simulink model "sldrt"  (R2018b)
settings: Solver=FixedStepAuto  StartTime=0.0  StopTime=Inf  FixedStep=1  RelTol=1e-3  EnableMultiTasking=on
values from neighbouring files (symbols this model uses):
  cpw = 4175    [symulacja.m]
  Cv01 = cpw*row*Vv    (= 801600)    [symulacja.m]
  Cv02 = cpw*row*Vv    (= 801600)    [symulacja.m]
  Cvg1 = cpw*row*Vg1    (= 400800)    [symulacja.m]
  Cvg2 = cpw*row*Vg2    (= 400800)    [symulacja.m]
  Cvs1 = cps*ros*Vs1    (= 38412000)    [symulacja.m]
  Cvs2 = cps*ros*Vs2    (= 38412000)    [symulacja.m]
  Cvw1 = cpp*rop*Vw1    (= 60000)    [symulacja.m]
  Cvw2 = cpp*rop*Vw2    (= 60000)    [symulacja.m]
  dfmw = 0    [symulacja.m]
  dTwz = 0    [symulacja.m]
  dTzew = 0    [symulacja.m]
  fmg1_0 = fmg1_N    (= 0.0239520958084)    [symulacja.m]
  fmg2_0 = fmg2_N    (= 0.0239520958084)    [symulacja.m]
  fmw0 = fmwN    (= 0.0479041916168)    [symulacja.m]
  Kcg1 = qg1_N/(Tgp1_N-Twew1_N)    (= 40)    [symulacja.m]
  Kcg2 = qg2_N/(Tgp2_N-Twew2_N)    (= 38.4615384615)    [symulacja.m]
  Kco = qwN/(TwpN-TozN)    (= 200)    [symulacja.m]
  Kcs1 = qg1_N/(Ts1_N-TzewN)    (= 80)    [symulacja.m]
  Kcs2 = qg2_N/(Ts2_N-TzewN)    (= 83.3333333333)    [symulacja.m]
  Kcw1 = qg1_N/(Twew1_N-Ts1_N)    (= 133.333333333)    [symulacja.m]
  Kcw2 = qg2_N/(Twew2_N-Ts2_N)    (= 142.857142857)    [symulacja.m]
  steptime = 1*czas/10^2    (= 30000)    [symulacja.m]
  Tdelay1 = 16000    [symulacja.m]
  Tdelay2 = Tdelay1    (= 16000)    [symulacja.m]
  Tgp1_0 = (C_1*Tgz1_0+Kcg1*Twew1_0)/(Kcg1+C_1)    (= 70)    [symulacja.m]
  Tgp2_0 = (C_2*Tgz2_0+Kcg2*Twew2_0)/(Kcg2+C_2)    (= 70)    [symulacja.m]
  Toz0 = (Kco*C1*Twz0+C2*(C1+Kco)*Top0)/M_1    (= 90)    [symulacja.m]
  Ts1_0 = (Kcw1*Twew1_0+Kcs1*Tzew0)/(Kcw1+Kcs1)    (= 5)    [symulacja.m]
  Ts2_0 = (Kcw2*Twew2_0+Kcs2*Tzew0)/(Kcw2+Kcs2)    (= 4)    [symulacja.m]
  Twew1_0 = (Kcg1*C_1*(Kcw1+Kcs1)*Tgz1_0+Kcw1*Kcs1*(Kcg1+C_1)*Tzew0)/M_1    (= 20)    [symulacja.m]
  Twew2_0 = (Kcg2*C_2*(Kcw2+Kcs2)*Tgz2_0+Kcw2*Kcs2*(Kcg2+C_2)*Tzew0)/M_2    (= 18)    [symulacja.m]
  Twp0 = (C1*Twz0+Kco*Toz0)/(C1+Kco)    (= 110)    [symulacja.m]
  Twz0 = TwzN    (= 130)    [symulacja.m]
  Tzew0 = TzewN    (= -20)    [symulacja.m]
libraries: sldrtlib x1
Description:
  | Water Tank Model with Dashboard
  | 
  | The example model "sldrtex_dashboard" shows a real-time model of a water tank
  | controlled by dashboard controls.  You can change the inputs to the plant using
  | the knobs and observe the response on the gauges.
  | 
  | How to run this model in Normal Mode:
  | 
  | 1) Double-click the orange button to switch to Normal Mode if needed.
  | 2) Start the real-time execution using Simulation->Run.
  | 3) Change the input flow and output valve values by the dashboard controls and observe
  |    the results on the dashboard gauges.
  | 
  | How to run this model in External Mode:
  | 
  | 1) Double-click the orange button to switch to External Mode if needed.
  | 2) Start the real-time execution using Simulation->Run. The model will automatically
  |    build, connect to Simulink in External Mode and start.
  | 3) Change the input flow and output valve values by the dashboard controls and observe
  |    the results on the dashboard gauges.
settings Model: EnablePacing=on  PacingRate=8000  ExtModeTrigDuration=101  Creator=The MathWorks, Inc.  LastModifiedBy=r3vus
settings DataIOCC: LimitDataPoints=on  SaveFormat=Array  SignalLoggingName=logsOut
settings OptimizationCC: ExpressionDepthLimit=2147483647  InitFltsAndDblsToZero=on  EfficientMapNaN2IntZero=off  LifeSpan=inf
settings DebuggingCC: UnderspecifiedInitializationDetection=Classic  MergeDetectMultiDrivingBlocksExec=none  SignalResolutionControl=TryResolveAllWithWarning  FcnCallInpInsideContextMsg=warning  AllowSymbolicDim=off  StateNameClashWarn=warning  SFUnexpectedBacktrackingDiag=warning  SFNoUnconditionalDefaultTransitionDiag=warning  SFExecutionAtInitializationDiag=none
settings HardwareCC: TargetBitPerLong=64  TargetBitPerPointer=64  TargetBitPerSizeT=64  TargetBitPerPtrDiffT=64  TargetIntDivRoundTo=Zero  TargetEndianess=LittleEndian  TargetWordSize=64  TargetHWDeviceType=Intel->x86-64
settings ModelReferenceCC: PropagateSignalLabelsOutOfModel=off
settings SFSimCC: SimUseLocalCustomCode=off
settings RTWCC: SystemTargetFile=sldrt.tlc  TemplateMakefile=sldrt.tmf  Description=Simulink Desktop Real-Time  RTWUseLocalCustomCode=off  RTWCompilerOptimization=on
settings CodeAppCC: MaxIdLength=95  StateflowObjectComments=on
settings SimulinkDesktopRealTimeCC: TargetPreCompLibLocation=D:\Program Files\MATLAB\R2018b\toolbox\sldrt\lib\win64  TargetLangStandard=C89/C90 (ANSI)  GeneratePreprocessorConditionals=Disable all  SupportVariableSizeSignals=off  PreserveStateflowLocalDataDimensions=off
settings ConfigComp: CovMetricSettings=dw  CovHtmlReporting=on  CovSaveCumulativeToWorkspaceVar=on  CovSaveSingleToWorkspaceVar=on  CovShowResultsExplorer=off  CovExternalEMLEnable=off  CovSFcnEnable=off

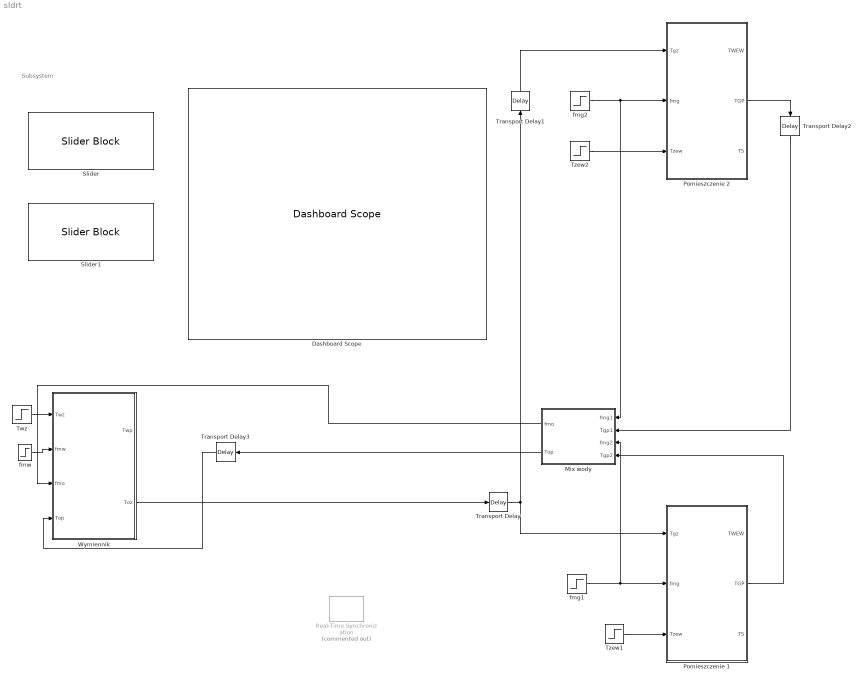
== system sldrt ==
  note: Subsystem
  Dashboard Scope : DashboardScope  WebBlockId=55  Ymin=10  Ymax=50
  Mix wody : Subsystem
  Pomieszczenie 1 : Subsystem  mask{Cvg=Cvg1, Cvs=Cvs1, Kcg=Kcg1, Kcw=Kcw1, cpw=cpw, Kcs=Kcs1, Cvw=Cvw1, Twew0=Twew1_0, Ts0=Ts1_0, Tgp0=Tgp1_0}
  Pomieszczenie 2 : Subsystem  mask{Cvg=Cvg2, Cvs=Cvs2, Kcg=Kcg2, Kcw=Kcw2, cpw=cpw, Kcs=Kcs2, Cvw=Cvw2, Twew0=Twew2_0, Ts0=Ts2_0, Tgp0=Tgp2_0}
  Real-Time Synchronization : sldrtlib/Real-Time Synchronization  Commented=on  SampleTime=1  MaxMissedTicks=10  ShowMissedTicks=off  YieldWhenWaiting=off
  Slider : SliderBlock  WebBlockId=118  ScaleMin=-20  ScaleMax=30
  Slider1 : SliderBlock  WebBlockId=119  ScaleMin=100  ScaleMax=130
  Transport Delay : TransportDelay  DelayTime=Tdelay1  InitialOutput=Toz0
  Transport Delay1 : TransportDelay  DelayTime=Tdelay2  InitialOutput=Toz0
  Transport Delay2 : TransportDelay  DelayTime=Tdelay2  InitialOutput=Tgp2_0
  Transport Delay3 : TransportDelay  DelayTime=Tdelay1  InitialOutput=(Tgp1_0*fmg1_0+Tgp2_0*fmg2_0)/(fmg1_0+fmg2_0)
  Twz : Step  Time=steptime  Before=Twz0  After=Twz0+dTwz  SampleTime=0
  Tzew1 : Step  Time=steptime  Before=Tzew0  After=Tzew0+dTzew  SampleTime=0
  Tzew2 : Step  Time=steptime  Before=Tzew0  After=Tzew0+dTzew  SampleTime=0
  Wymiennik : Subsystem
  fmg1 : Step  Time=steptime  Before=fmg1_0  After=fmg1_0  SampleTime=0
  fmg2 : Step  Time=steptime  Before=fmg2_0  After=fmg2_0  SampleTime=0
  fmw : Step  Time=steptime  Before=fmw0  After=fmw0+dfmw  SampleTime=0
  wires:
  Transport Delay1/1 -> Pomieszczenie 2/1(Tgz)
  Transport Delay3/1 -> Wymiennik/4(Top)
  Pomieszczenie 2/2(TGP) -> Transport Delay2/1
  Mix wody/1(fmo) -> Wymiennik/3(fmo)
  Transport Delay/1 -> Pomieszczenie 1/1(Tgz), Transport Delay1/1
  Mix wody/2(Top) -> Transport Delay3/1
  Wymiennik/2(Toz) -> Transport Delay/1
  fmg2/1 -> Mix wody/1(fmg1), Pomieszczenie 2/2(fmg)
  Twz/1 -> Wymiennik/1(Twz)
  Tzew1/1 -> Pomieszczenie 1/3(Tzew)
  Pomieszczenie 1/2(TGP) -> Mix wody/4(Tgp2)
  fmg1/1 -> Mix wody/3(fmg2), Pomieszczenie 1/2(fmg)
  Tzew2/1 -> Pomieszczenie 2/3(Tzew)
  fmw/1 -> Wymiennik/2(fmw)
  Transport Delay2/1 -> Mix wody/2(Tgp1)

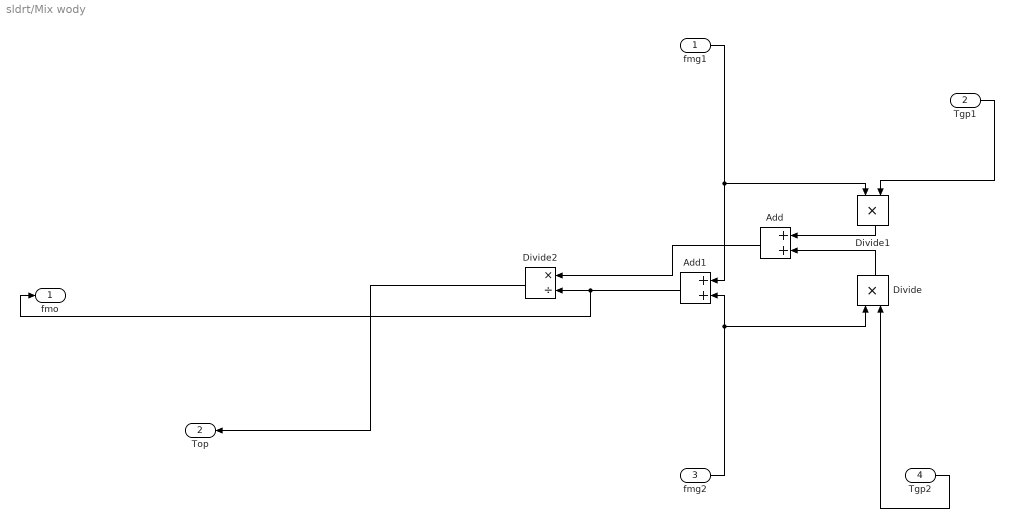
== system sldrt/Mix wody ==
  fmg1 : Inport
  Tgp1 : Inport  Port=2
  fmg2 : Inport  Port=3
  Tgp2 : Inport  Port=4
  Add : Sum
  Add1 : Sum
  Divide : Product  Inputs=**
  Divide1 : Product  Inputs=**
  Divide2 : Product  Inputs=*/
  fmo : Outport
  Top : Outport  Port=2
  wires:
  Tgp1/1 -> Divide1/2
  fmg2/1 -> Add1/2, Divide/1
  Divide/1 -> Add/2
  Add1/1 -> fmo/1, Divide2/2
  Tgp2/1 -> Divide/2
  fmg1/1 -> Add1/1, Divide1/1
  Divide1/1 -> Add/1
  Add/1 -> Divide2/1
  Divide2/1 -> Top/1

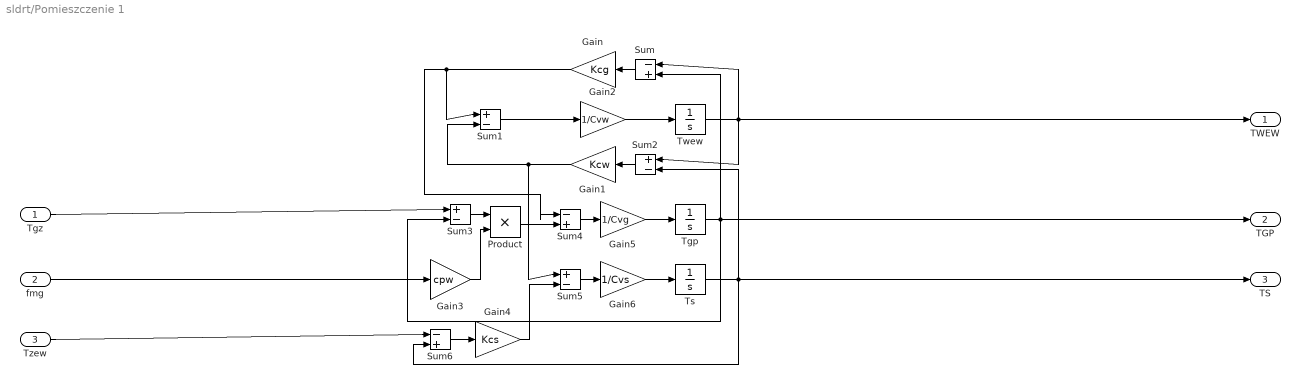
== system sldrt/Pomieszczenie 1 ==
  Tgz : Inport
  fmg : Inport  Port=2
  Tzew : Inport  Port=3
  Gain : Gain  Gain=Kcg
  Gain1 : Gain  Gain=Kcw
  Gain2 : Gain  Gain=1/Cvw
  Gain3 : Gain  Gain=cpw
  Gain4 : Gain  Gain=Kcs
  Gain5 : Gain  Gain=1/Cvg
  Gain6 : Gain  Gain=1/Cvs
  Product : Product
  Sum : Sum  Inputs=|-+
  Sum{1..3,5} (4 alike) : Sum  Inputs=|+-
  Sum4 : Sum  Inputs=|-+
  Sum6 : Sum  Inputs=|-+
  Tgp : Integrator  InitialCondition=Tgp0
  Ts : Integrator  InitialCondition=Ts0
  Twew : Integrator  InitialCondition=Twew0
  TWEW : Outport
  TGP : Outport  Port=2
  TS : Outport  Port=3
  wires:
  Twew/1 -> TWEW/1, Sum2/1, Sum/1
  Tgp/1 -> TGP/1, Sum3/2, Sum/2
  Sum/1 -> Gain/1
  Ts/1 -> TS/1, Sum6/2, Sum2/2
  Sum2/1 -> Gain1/1
  Gain1/1 -> Sum5/1, Sum1/2
  Sum1/1 -> Gain2/1
  Tgz/1 -> Sum3/1
  fmg/1 -> Gain3/1
  Gain3/1 -> Product/2
  Sum3/1 -> Product/1
  Gain/1 -> Sum1/1, Sum4/1
  Product/1 -> Sum4/2
  Sum4/1 -> Gain5/1
  Tzew/1 -> Sum6/1
  Sum6/1 -> Gain4/1
  Gain4/1 -> Sum5/2
  Sum5/1 -> Gain6/1
  Gain2/1 -> Twew/1
  Gain5/1 -> Tgp/1
  Gain6/1 -> Ts/1

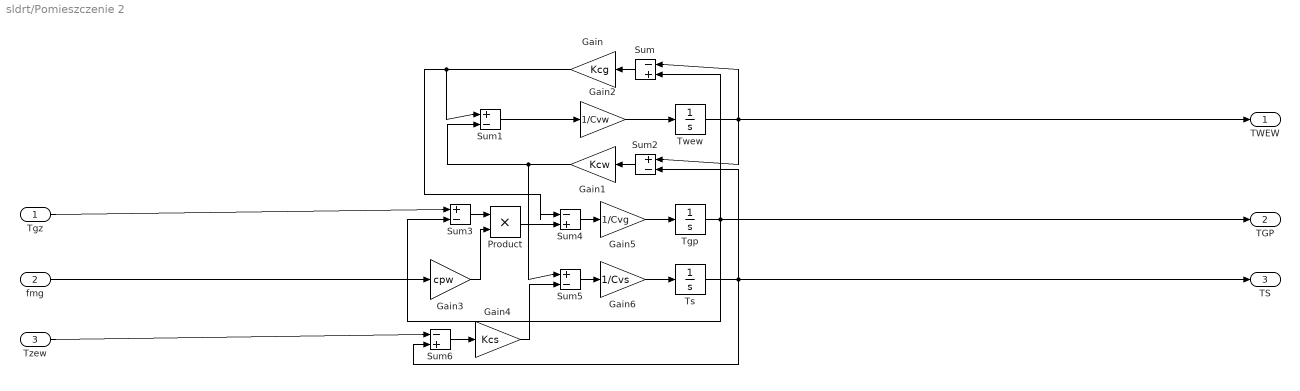
== system sldrt/Pomieszczenie 2 ==
  Tgz : Inport
  fmg : Inport  Port=2
  Tzew : Inport  Port=3
  Gain : Gain  Gain=Kcg
  Gain1 : Gain  Gain=Kcw
  Gain2 : Gain  Gain=1/Cvw
  Gain3 : Gain  Gain=cpw
  Gain4 : Gain  Gain=Kcs
  Gain5 : Gain  Gain=1/Cvg
  Gain6 : Gain  Gain=1/Cvs
  Product : Product
  Sum : Sum  Inputs=|-+
  Sum{1..3,5} (4 alike) : Sum  Inputs=|+-
  Sum4 : Sum  Inputs=|-+
  Sum6 : Sum  Inputs=|-+
  Tgp : Integrator  InitialCondition=Tgp0
  Ts : Integrator  InitialCondition=Ts0
  Twew : Integrator  InitialCondition=Twew0
  TWEW : Outport
  TGP : Outport  Port=2
  TS : Outport  Port=3
  wires:
  Twew/1 -> TWEW/1, Sum2/1, Sum/1
  Tgp/1 -> TGP/1, Sum3/2, Sum/2
  Sum/1 -> Gain/1
  Ts/1 -> TS/1, Sum6/2, Sum2/2
  Sum2/1 -> Gain1/1
  Gain1/1 -> Sum5/1, Sum1/2
  Sum1/1 -> Gain2/1
  Tgz/1 -> Sum3/1
  fmg/1 -> Gain3/1
  Gain3/1 -> Product/2
  Sum3/1 -> Product/1
  Gain/1 -> Sum1/1, Sum4/1
  Product/1 -> Sum4/2
  Sum4/1 -> Gain5/1
  Tzew/1 -> Sum6/1
  Sum6/1 -> Gain4/1
  Gain4/1 -> Sum5/2
  Sum5/1 -> Gain6/1
  Gain2/1 -> Twew/1
  Gain5/1 -> Tgp/1
  Gain6/1 -> Ts/1

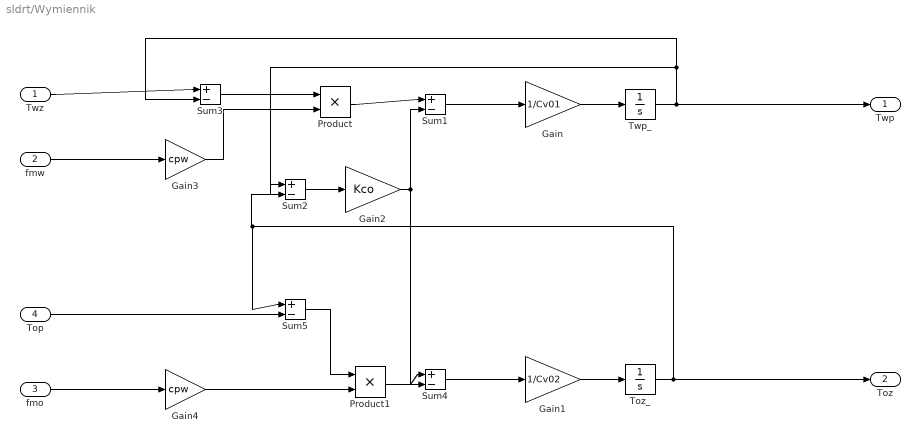
== system sldrt/Wymiennik ==
  Twz : Inport
  fmw : Inport  Port=2
  fmo : Inport  Port=3
  Top : Inport  Port=4
  Gain : Gain  Gain=1/Cv01
  Gain1 : Gain  Gain=1/Cv02
  Gain2 : Gain  Gain=Kco
  Gain3 : Gain  Gain=cpw
  Gain4 : Gain  Gain=cpw
  Product : Product
  Product1 : Product
  Sum{1..5} (5 alike) : Sum  Inputs=|+-
  Toz_ : Integrator  InitialCondition=Toz0
  Twp_ : Integrator  InitialCondition=Twp0
  Twp : Outport
  Toz : Outport  Port=2
  wires:
  Toz_/1 -> Sum5/1, Sum2/2, Toz/1
  Twp_/1 -> Sum2/1, Sum3/2, Twp/1
  Gain/1 -> Twp_/1
  Gain1/1 -> Toz_/1
  Gain3/1 -> Product/2
  fmw/1 -> Gain3/1
  Sum3/1 -> Product/1
  Twz/1 -> Sum3/1
  Product/1 -> Sum1/1
  Sum1/1 -> Gain/1
  Sum2/1 -> Gain2/1
  Sum4/1 -> Gain1/1
  Gain2/1 -> Sum1/2, Sum4/1
  fmo/1 -> Gain4/1
  Gain4/1 -> Product1/2
  Top/1 -> Sum5/2
  Sum5/1 -> Product1/1
  Product1/1 -> Sum4/2
